simulink model "SSIV_Simulink_Com"  (R2018a)
settings: Solver=FixedStepAuto  StartTime=0.0  StopTime=inf  FixedStep=.015  RelTol=1e-3  EnableMultiTasking=on
libraries: raspberrypilib x24, hdlsllib x21, simulink x11
(part 1 of 2)
settings Model: SimulationMode=external  Creator=domin  LastModifiedBy=domin
settings SolverCC: ConcurrentTasks=on  PositivePriorityOrder=on  AutoInsertRateTranBlk=on
settings DataIOCC: SaveFormat=Array
settings OptimizationCC: EnhancedBackFolding=on  PassReuseOutputArgsThreshold=0  MaxStackSize=64  OptimizeBlockOrder=speed  DifferentSizesBufferReuse=on  OptimizationCustomize=off
settings DebuggingCC: ParameterTunabilityLossMsg=error
settings HardwareCC: ProdBitPerPointer=32  ProdBitPerSizeT=32  ProdBitPerPtrDiffT=32  ProdLargestAtomicInteger=Long  ProdLargestAtomicFloat=Double  ProdWordSize=32  ProdHWDeviceType=ARM Compatible->ARM Cortex  UseEmbeddedCoderFeatures=off  UseSimulinkCoderFeatures=off
settings SFSimCC: MATLABDynamicMemAlloc=off
settings RTWCC: SystemTargetFile=ert.tlc  HardwareBoard=Raspberry Pi  TLCOptions="-aInlineSetEventsForThisBaseRateFcn=TLC_FALSE -aSuppressMultiTaskScheduler=TLC_FALSE  -aRateBasedStepFcn=0"  TemplateMakefile=ert_default_tmf  RTWVerbose=off  Toolchain=GNU GCC Raspberry Pi  BuildConfiguration=Faster Runs
settings CodeAppCC: ForceParamTrailComments=on  OperatorAnnotations=on  MangleLength=10
settings ERTTargetCC: ERTCustomFileBanners=off  SupportContinuousTime=on  SupportNonInlinedSFcns=on  RemoveResetFunc=off  SupportVariableSizeSignals=on  ModelStepFunctionPrototypeControlCompliant=off  ExtMode=on  ExtModeMexArgs='129.65.101.12' 0 17725  ERTSrcFileBannerTemplate=codertarget_code_template.cgt  ERTHdrFileBannerTemplate=codertarget_code_template.cgt  ERTDataSrcFileTemplate=codertarget_code_template.cgt  ERTDataHdrFileTemplate=codertarget_code_template.cgt

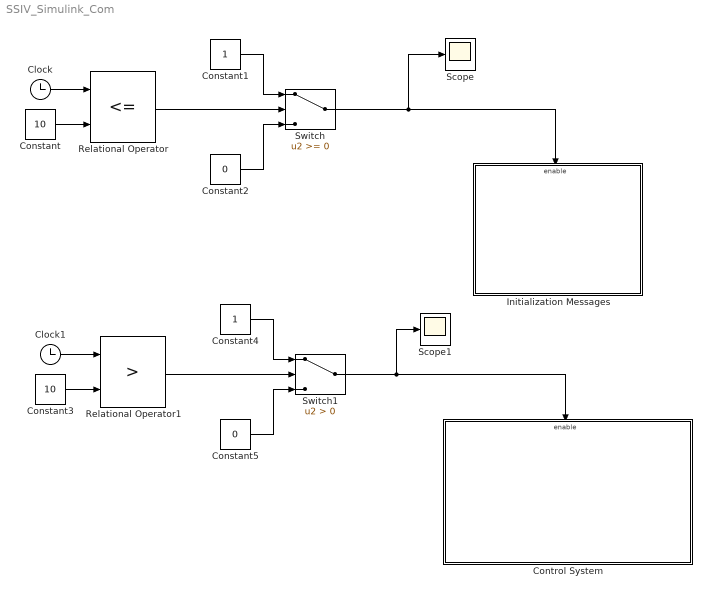
== system SSIV_Simulink_Com ==
  Clock : Clock
  Clock1 : Clock
  Constant : Constant  Value=10
  Constant1 : Constant
  Constant2 : Constant  Value=0
  Constant3 : Constant  Value=10
  Constant4 : Constant
  Constant5 : Constant  Value=0
  Control System : Subsystem
  Initialization Messages : Subsystem
  Relational Operator : RelationalOperator  Operator=<=  OutDataTypeStr=boolean  RndMeth=Simplest
  Relational Operator1 : RelationalOperator  Operator=>  OutDataTypeStr=boolean  RndMeth=Simplest
  Scope : Scope
  Scope1 : Scope
  Switch : Switch
  Switch1 : Switch  Criteria=u2 > Threshold
  wires:
  Clock/1 -> Relational Operator/1
  Constant/1 -> Relational Operator/2
  Relational Operator/1 -> Switch/2
  Constant1/1 -> Switch/1
  Constant2/1 -> Switch/3
  Switch/1 -> Scope/1, Initialization Messages/Enable
  Switch1/1 -> Scope1/1, Control System/Enable
  Constant5/1 -> Switch1/3
  Constant4/1 -> Switch1/1
  Relational Operator1/1 -> Switch1/2
  Constant3/1 -> Relational Operator1/2
  Clock1/1 -> Relational Operator1/1

== system SSIV_Simulink_Com/Control System ==
  Enable : EnablePort
  Const Mot Vel : Constant  Value=50
  SSIV Hardware Communication : Subsystem
  Throttle and Steering Handler : Subsystem
  wires:
  SSIV Hardware Communication/10(radio_throttle) -> Throttle and Steering Handler/1(Inport)
  SSIV Hardware Communication/11(radio_steering) -> Throttle and Steering Handler/3(Inport1)
  Throttle and Steering Handler/1(Throttle RF) -> SSIV Hardware Communication/1(throttle_right_front)
  Throttle and Steering Handler/2(Throttle LF) -> SSIV Hardware Communication/2(throttle_left_front)
  Throttle and Steering Handler/3(Throttle RR) -> SSIV Hardware Communication/3(throttle_right_rear)
  Throttle and Steering Handler/4(Throttle LR) -> SSIV Hardware Communication/4(throttle_left_rear)
  Throttle and Steering Handler/5(Outport) -> SSIV Hardware Communication/5(servo_out)
  Const Mot Vel/1 -> Throttle and Steering Handler/2(Inport2)

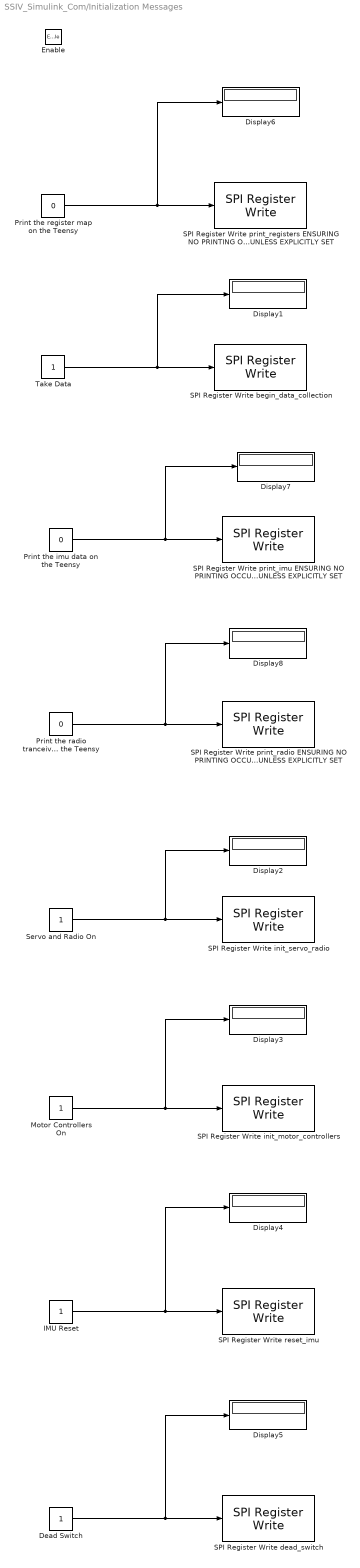
== system SSIV_Simulink_Com/Initialization Messages ==
  Enable : EnablePort
  Dead Switch : Constant  OutDataTypeStr=uint8
  Display{1..8} (8 alike) : Display
      settings: Format=decimal (Stored Integer)
  IMU Reset : Constant  OutDataTypeStr=uint8
  Motor Controllers On : Constant  OutDataTypeStr=uint8
  Print the imu data on the Teensy : Constant  Value=0  OutDataTypeStr=uint8
  Print the radio tranceiver data on the Teensy : Constant  Value=0  OutDataTypeStr=uint8
  Print the register map on the Teensy : Constant  Value=0  OutDataTypeStr=uint8
  SPI Register Write begin_data_collection : raspberrypilib/SPI Register Write  BoardProperty=Pi 3 Model B  SPIModule=uint32(0)  Mode=Master  BusSpeed=1000000  Pin=SPI0_CE1  FirstBitToTransfer=Most significant bit (MSB)  ClockMode=0  BlockFunction=Write  RegisterAddress=1  OutputDataType=int8  OutputDataLength=1
      settings: SourceProductName=Simulink Support Package for Raspberry Pi Hardware  SourceProductBaseCode=RASPPI
  SPI Register Write dead_switch : raspberrypilib/SPI Register Write  BoardProperty=Pi 3 Model B  SPIModule=uint32(0)  Mode=Master  BusSpeed=1000000  Pin=SPI0_CE1  FirstBitToTransfer=Most significant bit (MSB)  ClockMode=0  BlockFunction=Write  RegisterAddress=7  OutputDataType=int8  OutputDataLength=1
      settings: SourceProductName=Simulink Support Package for Raspberry Pi Hardware  SourceProductBaseCode=RASPPI
  SPI Register Write init_motor_controllers : raspberrypilib/SPI Register Write  BoardProperty=Pi 3 Model B  SPIModule=uint32(0)  Mode=Master  BusSpeed=1000000  Pin=SPI0_CE1  FirstBitToTransfer=Most significant bit (MSB)  ClockMode=0  BlockFunction=Write  RegisterAddress=5  OutputDataType=int8  OutputDataLength=1
      settings: SourceProductName=Simulink Support Package for Raspberry Pi Hardware  SourceProductBaseCode=RASPPI
  SPI Register Write init_servo_radio : raspberrypilib/SPI Register Write  BoardProperty=Pi 3 Model B  SPIModule=uint32(0)  Mode=Master  BusSpeed=1000000  Pin=SPI0_CE1  FirstBitToTransfer=Most significant bit (MSB)  ClockMode=0  BlockFunction=Write  RegisterAddress=4  OutputDataType=int8  OutputDataLength=1
      settings: SourceProductName=Simulink Support Package for Raspberry Pi Hardware  SourceProductBaseCode=RASPPI
  SPI Register Write print_imu ENSURING NO PRINTING OCCURS DURING DYNAMIC OP UNLESS EXPLICITLY SET : raspberrypilib/SPI Register Write  BoardProperty=Pi 3 Model B  SPIModule=uint32(0)  Mode=Master  BusSpeed=1000000  Pin=SPI0_CE1  FirstBitToTransfer=Most significant bit (MSB)  ClockMode=0  BlockFunction=Write  RegisterAddress=2  OutputDataType=int8  OutputDataLength=1
      settings: SourceProductName=Simulink Support Package for Raspberry Pi Hardware  SourceProductBaseCode=RASPPI
  SPI Register Write print_radio ENSURING NO PRINTING OCCURS DURING DYNAMIC OP UNLESS EXPLICITLY SET : raspberrypilib/SPI Register Write  BoardProperty=Pi 3 Model B  SPIModule=uint32(0)  Mode=Master  BusSpeed=1000000  Pin=SPI0_CE1  FirstBitToTransfer=Most significant bit (MSB)  ClockMode=0  BlockFunction=Write  RegisterAddress=3  OutputDataType=int8  OutputDataLength=1
      settings: SourceProductName=Simulink Support Package for Raspberry Pi Hardware  SourceProductBaseCode=RASPPI
  SPI Register Write print_registers ENSURING NO PRINTING OCCURS DURING DYNAMIC OP UNLESS EXPLICITLY SET : raspberrypilib/SPI Register Write  BoardProperty=Pi 3 Model B  SPIModule=uint32(0)  Mode=Master  BusSpeed=1000000  Pin=SPI0_CE1  FirstBitToTransfer=Most significant bit (MSB)  ClockMode=0  BlockFunction=Write  RegisterAddress=0  OutputDataType=int8  OutputDataLength=1
      settings: SourceProductName=Simulink Support Package for Raspberry Pi Hardware  SourceProductBaseCode=RASPPI
  SPI Register Write reset_imu : raspberrypilib/SPI Register Write  BoardProperty=Pi 3 Model B  SPIModule=uint32(0)  Mode=Master  BusSpeed=1000000  Pin=SPI0_CE1  FirstBitToTransfer=Most significant bit (MSB)  ClockMode=0  BlockFunction=Write  RegisterAddress=6  OutputDataType=int8  OutputDataLength=1
      settings: SourceProductName=Simulink Support Package for Raspberry Pi Hardware  SourceProductBaseCode=RASPPI
  Servo and Radio On : Constant  OutDataTypeStr=uint8
  Take Data : Constant  OutDataTypeStr=uint8
  wires:
  Take Data/1 -> Display1/1, SPI Register Write begin_data_collection/1
  Servo and Radio On/1 -> SPI Register Write init_servo_radio/1, Display2/1
  Motor Controllers On/1 -> Display3/1, SPI Register Write init_motor_controllers/1
  IMU Reset/1 -> SPI Register Write reset_imu/1, Display4/1
  Dead Switch/1 -> Display5/1, SPI Register Write dead_switch/1
  Print the register map on the Teensy/1 -> SPI Register Write print_registers ENSURING NO PRINTING OCCURS DURING DYNAMIC OP UNLESS EXPLICITLY SET/1, Display6/1
  Print the imu data on the Teensy/1 -> SPI Register Write print_imu ENSURING NO PRINTING OCCURS DURING DYNAMIC OP UNLESS EXPLICITLY SET/1, Display7/1
  Print the radio tranceiver data on the Teensy/1 -> Display8/1, SPI Register Write print_radio ENSURING NO PRINTING OCCURS DURING DYNAMIC OP UNLESS EXPLICITLY SET/1

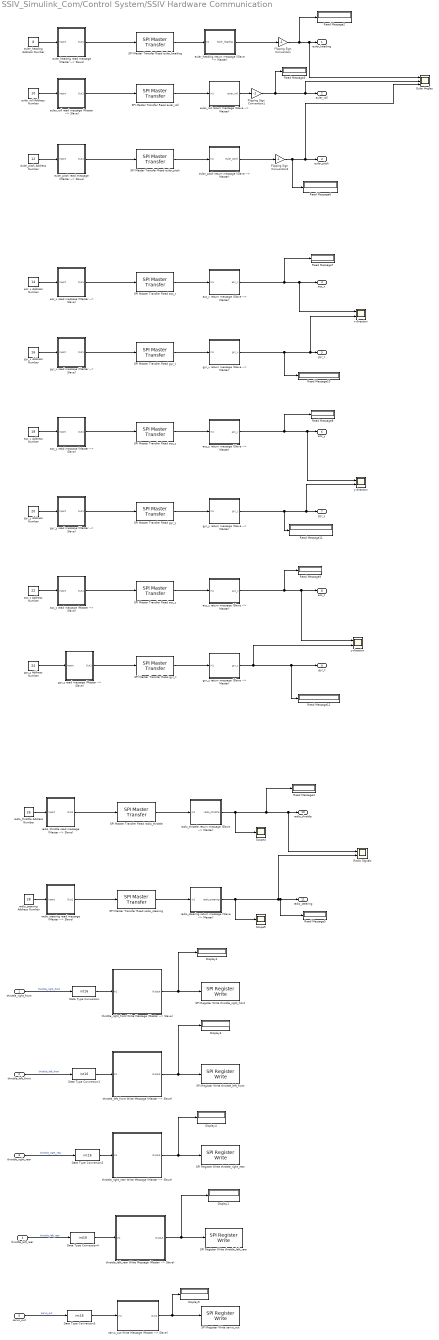
== system SSIV_Simulink_Com/Control System/SSIV Hardware Communication ==
  throttle_right_front : Inport
  throttle_left_front : Inport  Port=2
  throttle_right_rear : Inport  Port=3
  throttle_left_rear : Inport  Port=4
  servo_out : Inport  Port=5
  Data Type Conversion{,1..4} (5 alike) : DataTypeConversion  OutDataTypeStr=int16  RndMeth=Nearest
  Display{1..5} (5 alike) : Display
      settings: Format=decimal (Stored Integer)
  Euler Angles : Scope  NumInputPorts=3
  Flipping Sign Convention : Gain  Gain=-1
  Flipping Sign Convention1 : Gain  Gain=-1
  Flipping Sign Convention2 : Gain  Gain=-1
  Radio SIgnals : Scope  NumInputPorts=2
  Read Message{2..12} (11 alike) : Display
      settings: Format=decimal (Stored Integer)
  SPI Master Transfer Read acc_x : raspberrypilib/SPI Master Transfer  BoardProperty=Pi 3 Model B  SPIModule=uint32(0)  Mode=Master  BusSpeed=1000000  Pin=SPI0_CE1  FirstBitToTransfer=Most significant bit (MSB)  ClockMode=0  BlockFunction=Transfer  RegisterAddress=0  OutputDataType=int8  OutputDataLength=1
      settings: SourceProductName=Simulink Support Package for Raspberry Pi Hardware  SourceProductBaseCode=RASPPI
  SPI Master Transfer Read acc_y : raspberrypilib/SPI Master Transfer  BoardProperty=Pi 3 Model B  SPIModule=uint32(0)  Mode=Master  BusSpeed=1000000  Pin=SPI0_CE1  FirstBitToTransfer=Most significant bit (MSB)  ClockMode=0  BlockFunction=Transfer  RegisterAddress=0  OutputDataType=int8  OutputDataLength=1
      settings: SourceProductName=Simulink Support Package for Raspberry Pi Hardware  SourceProductBaseCode=RASPPI
  SPI Master Transfer Read acc_z : raspberrypilib/SPI Master Transfer  BoardProperty=Pi 3 Model B  SPIModule=uint32(0)  Mode=Master  BusSpeed=1000000  Pin=SPI0_CE1  FirstBitToTransfer=Most significant bit (MSB)  ClockMode=0  BlockFunction=Transfer  RegisterAddress=0  OutputDataType=int8  OutputDataLength=1
      settings: SourceProductName=Simulink Support Package for Raspberry Pi Hardware  SourceProductBaseCode=RASPPI
  SPI Master Transfer Read euler_heading : raspberrypilib/SPI Master Transfer  BoardProperty=Pi 3 Model B  SPIModule=uint32(0)  Mode=Master  BusSpeed=1000000  Pin=SPI0_CE1  FirstBitToTransfer=Most significant bit (MSB)  ClockMode=0  BlockFunction=Transfer  RegisterAddress=0  OutputDataType=int8  OutputDataLength=1
      settings: SourceProductName=Simulink Support Package for Raspberry Pi Hardware  SourceProductBaseCode=RASPPI
  SPI Master Transfer Read euler_pitch : raspberrypilib/SPI Master Transfer  BoardProperty=Pi 3 Model B  SPIModule=uint32(0)  Mode=Master  BusSpeed=1000000  Pin=SPI0_CE1  FirstBitToTransfer=Most significant bit (MSB)  ClockMode=0  BlockFunction=Transfer  RegisterAddress=0  OutputDataType=int8  OutputDataLength=1
      settings: SourceProductName=Simulink Support Package for Raspberry Pi Hardware  SourceProductBaseCode=RASPPI
  SPI Master Transfer Read euler_roll : raspberrypilib/SPI Master Transfer  BoardProperty=Pi 3 Model B  SPIModule=uint32(0)  Mode=Master  BusSpeed=1000000  Pin=SPI0_CE1  FirstBitToTransfer=Most significant bit (MSB)  ClockMode=0  BlockFunction=Transfer  RegisterAddress=0  OutputDataType=int8  OutputDataLength=1
      settings: SourceProductName=Simulink Support Package for Raspberry Pi Hardware  SourceProductBaseCode=RASPPI
  SPI Master Transfer Read gyr_x : raspberrypilib/SPI Master Transfer  BoardProperty=Pi 3 Model B  SPIModule=uint32(0)  Mode=Master  BusSpeed=1000000  Pin=SPI0_CE1  FirstBitToTransfer=Most significant bit (MSB)  ClockMode=0  BlockFunction=Transfer  RegisterAddress=0  OutputDataType=int8  OutputDataLength=1
      settings: SourceProductName=Simulink Support Package for Raspberry Pi Hardware  SourceProductBaseCode=RASPPI
  SPI Master Transfer Read gyr_y : raspberrypilib/SPI Master Transfer  BoardProperty=Pi 3 Model B  SPIModule=uint32(0)  Mode=Master  BusSpeed=1000000  Pin=SPI0_CE1  FirstBitToTransfer=Most significant bit (MSB)  ClockMode=0  BlockFunction=Transfer  RegisterAddress=0  OutputDataType=int8  OutputDataLength=1
      settings: SourceProductName=Simulink Support Package for Raspberry Pi Hardware  SourceProductBaseCode=RASPPI
  SPI Master Transfer Read gyr_z : raspberrypilib/SPI Master Transfer  BoardProperty=Pi 3 Model B  SPIModule=uint32(0)  Mode=Master  BusSpeed=1000000  Pin=SPI0_CE1  FirstBitToTransfer=Most significant bit (MSB)  ClockMode=0  BlockFunction=Transfer  RegisterAddress=0  OutputDataType=int8  OutputDataLength=1
      settings: SourceProductName=Simulink Support Package for Raspberry Pi Hardware  SourceProductBaseCode=RASPPI
  SPI Master Transfer Read radio_steering : raspberrypilib/SPI Master Transfer  BoardProperty=Pi 3 Model B  SPIModule=uint32(0)  Mode=Master  BusSpeed=1000000  Pin=SPI0_CE1  FirstBitToTransfer=Most significant bit (MSB)  ClockMode=0  BlockFunction=Transfer  RegisterAddress=0  OutputDataType=int8  OutputDataLength=1
      settings: SourceProductName=Simulink Support Package for Raspberry Pi Hardware  SourceProductBaseCode=RASPPI
  SPI Master Transfer Read radio_throttle : raspberrypilib/SPI Master Transfer  BoardProperty=Pi 3 Model B  SPIModule=uint32(0)  Mode=Master  BusSpeed=1000000  Pin=SPI0_CE1  FirstBitToTransfer=Most significant bit (MSB)  ClockMode=0  BlockFunction=Transfer  RegisterAddress=0  OutputDataType=int8  OutputDataLength=1
      settings: SourceProductName=Simulink Support Package for Raspberry Pi Hardware  SourceProductBaseCode=RASPPI
  "SPI Register Write servo_out " : raspberrypilib/SPI Register Write  BoardProperty=Pi 3 Model B  SPIModule=uint32(0)  Mode=Master  BusSpeed=1000000  Pin=SPI0_CE1  FirstBitToTransfer=Most significant bit (MSB)  ClockMode=0  BlockFunction=Write  RegisterAddress=38  OutputDataType=int8  OutputDataLength=1
      settings: SourceProductName=Simulink Support Package for Raspberry Pi Hardware  SourceProductBaseCode=RASPPI
  SPI Register Write throttle_left_front : raspberrypilib/SPI Register Write  BoardProperty=Pi 3 Model B  SPIModule=uint32(0)  Mode=Master  BusSpeed=1000000  Pin=SPI0_CE1  FirstBitToTransfer=Most significant bit (MSB)  ClockMode=0  BlockFunction=Write  RegisterAddress=32  OutputDataType=int8  OutputDataLength=1
      settings: SourceProductName=Simulink Support Package for Raspberry Pi Hardware  SourceProductBaseCode=RASPPI
  SPI Register Write throttle_left_rear : raspberrypilib/SPI Register Write  BoardProperty=Pi 3 Model B  SPIModule=uint32(0)  Mode=Master  BusSpeed=1000000  Pin=SPI0_CE1  FirstBitToTransfer=Most significant bit (MSB)  ClockMode=0  BlockFunction=Write  RegisterAddress=36  OutputDataType=int8  OutputDataLength=1
      settings: SourceProductName=Simulink Support Package for Raspberry Pi Hardware  SourceProductBaseCode=RASPPI
  SPI Register Write throttle_right_front : raspberrypilib/SPI Register Write  BoardProperty=Pi 3 Model B  SPIModule=uint32(0)  Mode=Master  BusSpeed=1000000  Pin=SPI0_CE1  FirstBitToTransfer=Most significant bit (MSB)  ClockMode=0  BlockFunction=Write  RegisterAddress=30  OutputDataType=int8  OutputDataLength=1
      settings: SourceProductName=Simulink Support Package for Raspberry Pi Hardware  SourceProductBaseCode=RASPPI
  SPI Register Write throttle_right_rear : raspberrypilib/SPI Register Write  BoardProperty=Pi 3 Model B  SPIModule=uint32(0)  Mode=Master  BusSpeed=1000000  Pin=SPI0_CE1  FirstBitToTransfer=Most significant bit (MSB)  ClockMode=0  BlockFunction=Write  RegisterAddress=34  OutputDataType=int8  OutputDataLength=1
      settings: SourceProductName=Simulink Support Package for Raspberry Pi Hardware  SourceProductBaseCode=RASPPI
  Scope4 : Scope
  Scope5 : Scope
  acc_x Address Number : Constant  Value=14  OutDataTypeStr=uint8
  acc_x read message (Master --> Slave) : Subsystem
  acc_x return message (Slave --> Master) : Subsystem
  acc_y Address Number : Constant  Value=18  OutDataTypeStr=uint8
  acc_y read message (Master --> Slave) : Subsystem
  acc_y return message (Slave --> Master) : Subsystem
  acc_z Address Number : Constant  Value=22  OutDataTypeStr=uint8
  acc_z read message (Master --> Slave) : Subsystem
  acc_z return message (Slave --> Master) : Subsystem
  euler_heading Address Number : Constant  Value=8  OutDataTypeStr=uint8
  euler_heading read message (Master --> Slave) : Subsystem
  euler_heading return message (Slave --> Master) : Subsystem
  euler_pitch Address Number : Constant  Value=12  OutDataTypeStr=uint8
  euler_pitch read message (Master --> Slave) : Subsystem
  euler_pitch return message (Slave --> Master) : Subsystem
  euler_roll Address Number : Constant  Value=10  OutDataTypeStr=uint8
  euler_roll read message (Master --> Slave) : Subsystem
  euler_roll return message (Slave --> Master) : Subsystem
  gyr_x Address Number : Constant  Value=16  OutDataTypeStr=uint8
  gyr_x read message (Master --> Slave) : Subsystem
  gyr_x return message (Slave --> Master) : Subsystem
  "gyr_y Address Number " : Constant  Value=20  OutDataTypeStr=uint8
  gyr_y read message (Master --> Slave) : Subsystem
  gyr_y return message (Slave --> Master) : Subsystem
  gyr_z Address Number : Constant  Value=24  OutDataTypeStr=uint8
  gyr_z read message (Master --> Slave) : Subsystem
  gyr_z return message (Slave --> Master) : Subsystem
  radio_steering Address Number : Constant  Value=28  OutDataTypeStr=uint8
  radio_steering read message (Master --> Slave) : Subsystem
  radio_steering return message (Slave --> Master) : Subsystem
  "radio_throttle Address Number " : Constant  Value=26  OutDataTypeStr=uint8
  radio_throttle read message (Master --> Slave) : Subsystem
  radio_throttle return message (Slave --> Master) : Subsystem
  servo_out Write Message (Master --> Slave) : Subsystem
  throttle_left_front Write Message (Master --> Slave) : Subsystem
  throttle_left_rear Write Message (Master --> Slave) : Subsystem
  throttle_right_front Write Message (Master --> Slave) : Subsystem
  throttle_right_rear Write Message (Master --> Slave) : Subsystem
  x-direction : Scope  NumInputPorts=2
  y-direction : Scope  NumInputPorts=2
  z-direction : Scope  NumInputPorts=2
  euler_heading : Outport
  euler_roll : Outport  Port=2
  euler_pitch : Outport  Port=3
  acc_x : Outport  Port=4
  gyr_x : Outport  Port=5
  acc_y : Outport  Port=6
  gyr_y : Outport  Port=7
  acc_z : Outport  Port=8
  gyr_z : Outport  Port=9
  radio_throttle : Outport  Port=10
  radio_steering : Outport  Port=11
  wires:
  euler_heading read message (Master --> Slave)/1(Out1) -> SPI Master Transfer Read euler_heading/1
  euler_heading return message (Slave --> Master)/1(euler_heading) -> Flipping Sign Convention/1
  SPI Master Transfer Read euler_heading/1 -> euler_heading return message (Slave --> Master)/1(In1)
  throttle_left_rear Write Message (Master --> Slave)/1(Output) -> Display1/1, SPI Register Write throttle_left_rear/1
  throttle_left_rear/1 -> Data Type Conversion4/1  "throttle_left_rear"
  SPI Master Transfer Read radio_throttle/1 -> radio_throttle return message (Slave --> Master)/1(In1)
  radio_throttle read message (Master --> Slave)/1(Out1) -> SPI Master Transfer Read radio_throttle/1
  radio_throttle return message (Slave --> Master)/1(radio_throttle) -> Read Message4/1, Radio SIgnals/1, radio_throttle/1, Scope4/1
  radio_steering return message (Slave --> Master)/1(radio_steering) -> Read Message5/1, radio_steering/1, Radio SIgnals/2, Scope5/1
  radio_steering read message (Master --> Slave)/1(Out1) -> SPI Master Transfer Read radio_steering/1
  SPI Master Transfer Read radio_steering/1 -> radio_steering return message (Slave --> Master)/1(In1)
  servo_out/1 -> Data Type Conversion3/1  "servo_out"
  servo_out Write Message (Master --> Slave)/1(Out1) -> Display5/1, "SPI Register Write servo_out "/1
  acc_x return message (Slave --> Master)/1(acc_x) -> Read Message7/1, x-direction/1, acc_x/1
  SPI Master Transfer Read acc_x/1 -> acc_x return message (Slave --> Master)/1(In1)
  acc_x read message (Master --> Slave)/1(Out1) -> SPI Master Transfer Read acc_x/1
  acc_y read message (Master --> Slave)/1(Out1) -> SPI Master Transfer Read acc_y/1
  SPI Master Transfer Read acc_y/1 -> acc_y return message (Slave --> Master)/1(In1)
  acc_y return message (Slave --> Master)/1(acc_y) -> y-direction/1, acc_y/1, Read Message8/1
  acc_z return message (Slave --> Master)/1(acc_z) -> z-direction/1, acc_z/1, Read Message9/1
  SPI Master Transfer Read acc_z/1 -> acc_z return message (Slave --> Master)/1(In1)
  acc_z read message (Master --> Slave)/1(Out1) -> SPI Master Transfer Read acc_z/1
  gyr_z read message (Master --> Slave)/1(Out1) -> SPI Master Transfer Read gyr_z/1
  SPI Master Transfer Read gyr_z/1 -> gyr_z return message (Slave --> Master)/1(In1)
  gyr_z return message (Slave --> Master)/1(gyr_z) -> z-direction/2, gyr_z/1, Read Message12/1
  gyr_y return message (Slave --> Master)/1(gyr_y) -> Read Message11/1, y-direction/2, gyr_y/1
  SPI Master Transfer Read gyr_y/1 -> gyr_y return message (Slave --> Master)/1(In1)
  gyr_y read message (Master --> Slave)/1(Out1) -> SPI Master Transfer Read gyr_y/1
  gyr_x read message (Master --> Slave)/1(Out1) -> SPI Master Transfer Read gyr_x/1
  SPI Master Transfer Read gyr_x/1 -> gyr_x return message (Slave --> Master)/1(In1)
  gyr_x return message (Slave --> Master)/1(gyr_x) -> x-direction/2, gyr_x/1, Read Message10/1
  throttle_right_front/1 -> Data Type Conversion/1  "throttle_right_front"
  throttle_right_front Write Message (Master --> Slave)/1(Output) -> SPI Register Write throttle_right_front/1, Display2/1
  throttle_right_rear Write Message (Master --> Slave)/1(Output) -> Display4/1, SPI Register Write throttle_right_rear/1
  throttle_right_rear/1 -> Data Type Conversion2/1  "throttle_right_rear"
  throttle_left_front/1 -> Data Type Conversion1/1  "throttle_left_front"
  throttle_left_front Write Message (Master --> Slave)/1(Output) -> SPI Register Write throttle_left_front/1, Display3/1
  Data Type Conversion/1 -> throttle_right_front Write Message (Master --> Slave)/1(In1)
  Data Type Conversion1/1 -> throttle_left_front Write Message (Master --> Slave)/1(In1)
  Data Type Conversion2/1 -> throttle_right_rear Write Message (Master --> Slave)/1(In1)
  Data Type Conversion3/1 -> servo_out Write Message (Master --> Slave)/1(In1)
  Data Type Conversion4/1 -> throttle_left_rear Write Message (Master --> Slave)/1(In1)
  "radio_throttle Address Number "/1 -> radio_throttle read message (Master --> Slave)/1(Inport)
  gyr_z Address Number/1 -> gyr_z read message (Master --> Slave)/1(Inport)
  "gyr_y Address Number "/1 -> gyr_y read message (Master --> Slave)/1(Inport)
  gyr_x Address Number/1 -> gyr_x read message (Master --> Slave)/1(Inport)
  acc_z Address Number/1 -> acc_z read message (Master --> Slave)/1(Inport)
  acc_y Address Number/1 -> acc_y read message (Master --> Slave)/1(Inport)
  acc_x Address Number/1 -> acc_x read message (Master --> Slave)/1(Inport)
  euler_heading Address Number/1 -> euler_heading read message (Master --> Slave)/1(Inport)
  radio_steering Address Number/1 -> radio_steering read message (Master --> Slave)/1(Inport)
  SPI Master Transfer Read euler_roll/1 -> euler_roll return message (Slave --> Master)/1(In1)
  euler_roll Address Number/1 -> euler_roll read message (Master --> Slave)/1(Inport)
  euler_roll read message (Master --> Slave)/1(Out1) -> SPI Master Transfer Read euler_roll/1
  euler_roll return message (Slave --> Master)/1(euler_roll) -> Flipping Sign Convention1/1
  euler_pitch return message (Slave --> Master)/1(euler_pitch) -> Flipping Sign Convention2/1
  euler_pitch Address Number/1 -> euler_pitch read message (Master --> Slave)/1(Inport)
  SPI Master Transfer Read euler_pitch/1 -> euler_pitch return message (Slave --> Master)/1(In1)
  euler_pitch read message (Master --> Slave)/1(Out1) -> SPI Master Transfer Read euler_pitch/1
  Flipping Sign Convention/1 -> Read Message2/1, Euler Angles/1, euler_heading/1
  Flipping Sign Convention1/1 -> Read Message3/1, Euler Angles/2, euler_roll/1
  Flipping Sign Convention2/1 -> Read Message6/1, Euler Angles/3, euler_pitch/1

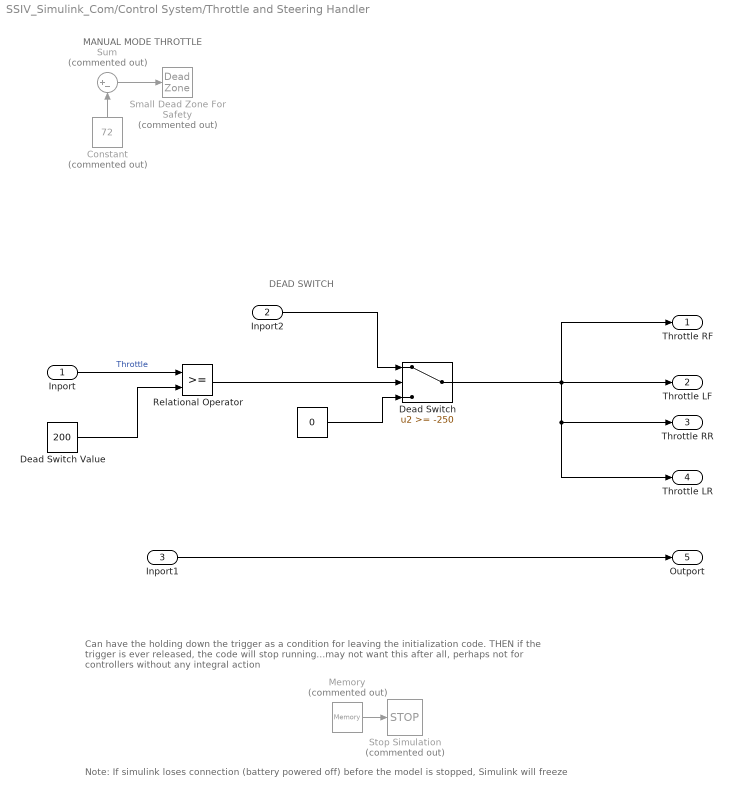
== system SSIV_Simulink_Com/Control System/Throttle and Steering Handler ==
  note: MANUAL MODE THROTTLE
  note: DEAD SWITCH
  note: Note: If simulink loses connection (battery powered off) before the model is stopped, Simulink will freeze
  note: Can have the holding down the trigger as a condition for leaving the initialization code. THEN if the trigger is ever released, the code will stop running...may not want this after all, perhaps not for controllers without any integral action
  Inport : Inport
  Inport2 : Inport  Port=2
  Inport1 : Inport  Port=3
  " " : Constant  Value=0
  Constant : Constant  Commented=on  Value=72
  Dead Switch : Switch  Threshold=-250
  Dead Switch Value : Constant  Value=200
  Memory : Memory  Commented=on
  Relational Operator : RelationalOperator  RndMeth=Simplest
  Small Dead Zone For Safety : DeadZone  Commented=on  LowerValue=-10  UpperValue=10
  Stop Simulation : Stop  Commented=on
  Sum : Sum  Commented=on  Inputs=|+-
  Throttle RF : Outport
  Throttle LF : Outport  Port=2
  Throttle RR : Outport  Port=3
  Throttle LR : Outport  Port=4
  Outport : Outport  Port=5
  wires:
  Inport1/1 -> Outport/1
  " "/1 -> Dead Switch/3
  Inport2/1 -> Dead Switch/1
  Relational Operator/1 -> Dead Switch/2
  Dead Switch/1 -> Throttle LF/1, Throttle LR/1, Throttle RR/1, Throttle RF/1
  Inport/1 -> Relational Operator/1  "Throttle"
  Memory/1 -> Stop Simulation/1
  Dead Switch Value/1 -> Relational Operator/2
  Constant/1 -> Sum/2
  Sum/1 -> Small Dead Zone For Safety/1

== system SSIV_Simulink_Com/Control System/SSIV Hardware Communication/acc_x read message (Master --> Slave) ==
  Inport : Inport
  Mux : Mux
      settings: DisplayOption=signals
  Read Bit Set : simulink/Logic and Bit Operations/Bit Set  iBit=7
      settings: SourceProductName=Simulink  SourceProductBaseCode=SL
  uint8_t 1 : Constant  OutDataTypeStr=uint8
  uint8_t 2 : Constant  OutDataTypeStr=uint8
  uint8_t 3 : Constant  OutDataTypeStr=uint8
  Out1 : Outport
  wires:
  Read Bit Set/1 -> Mux/1  "Addres/RW Byte acc_x Teensy Status will be returned here"
  uint8_t 1/1 -> Mux/2  "Junk will be returned here"
  Inport/1 -> Read Bit Set/1
  uint8_t 3/1 -> Mux/4  "Byte 1 will be returned here"
  Mux/1 -> Out1/1
  uint8_t 2/1 -> Mux/3  "Byte 0 will be returned here"

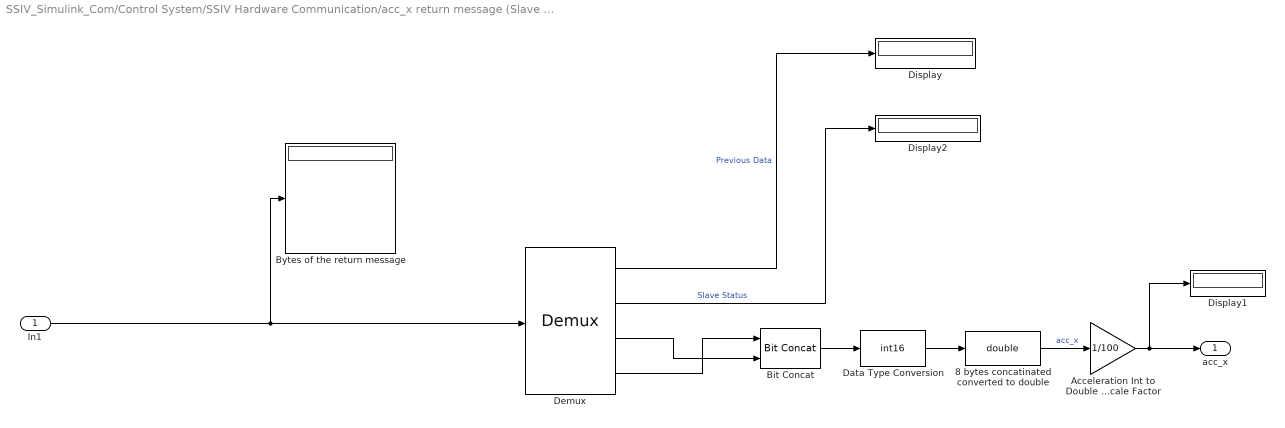
== system SSIV_Simulink_Com/Control System/SSIV Hardware Communication/acc_x return message (Slave --> Master) ==
  In1 : Inport
  8 bytes concatinated converted to double : DataTypeConversion  OutDataTypeStr=double  RndMeth=Nearest
  Acceleration Int to Double Scale Factor : Gain  Gain=1/100
  Bit Concat : hdlsllib/Logic and Bit Operations/Bit Concat  numInputs=2
      settings: SourceProductName=HDL Coder  SourceProductBaseCode=HD
  Bytes of the return message : Display
      settings: Format=decimal (Stored Integer)
  Data Type Conversion : DataTypeConversion  OutDataTypeStr=int16  RndMeth=Nearest
  Demux : Demux
  Display : Display
      settings: Format=binary (Stored Integer)
  Display1 : Display
      settings: Format=decimal (Stored Integer)
  Display2 : Display
      settings: Format=binary (Stored Integer)
  acc_x : Outport
  wires:
  8 bytes concatinated converted to double/1 -> Acceleration Int to Double Scale Factor/1  "acc_x"
  Demux/2 -> Display2/1  "Slave Status"
  Demux/1 -> Display/1  "Previous Data"
  In1/1 -> Bytes of the return message/1, Demux/1
  Bit Concat/1 -> Data Type Conversion/1
  Demux/4 -> Bit Concat/1
  Demux/3 -> Bit Concat/2
  Acceleration Int to Double Scale Factor/1 -> Display1/1, acc_x/1
  Data Type Conversion/1 -> 8 bytes concatinated converted to double/1

== system SSIV_Simulink_Com/Control System/SSIV Hardware Communication/acc_y read message (Master --> Slave) ==
  Inport : Inport
  Mux : Mux
      settings: DisplayOption=signals
  Read Bit Set : simulink/Logic and Bit Operations/Bit Set  iBit=7
      settings: SourceProductName=Simulink  SourceProductBaseCode=SL
  uint8_t 1 : Constant  OutDataTypeStr=uint8
  uint8_t 2 : Constant  OutDataTypeStr=uint8
  uint8_t 3 : Constant  OutDataTypeStr=uint8
  Out1 : Outport
  wires:
  uint8_t 2/1 -> Mux/3  "Byte 0 will be returned here"
  Mux/1 -> Out1/1
  uint8_t 3/1 -> Mux/4  "Byte 1 will be returned here"
  Inport/1 -> Read Bit Set/1
  uint8_t 1/1 -> Mux/2  "Junk will be returned here"
  Read Bit Set/1 -> Mux/1  "Addres/RW Byte acc_y Teensy Status will be returned here"

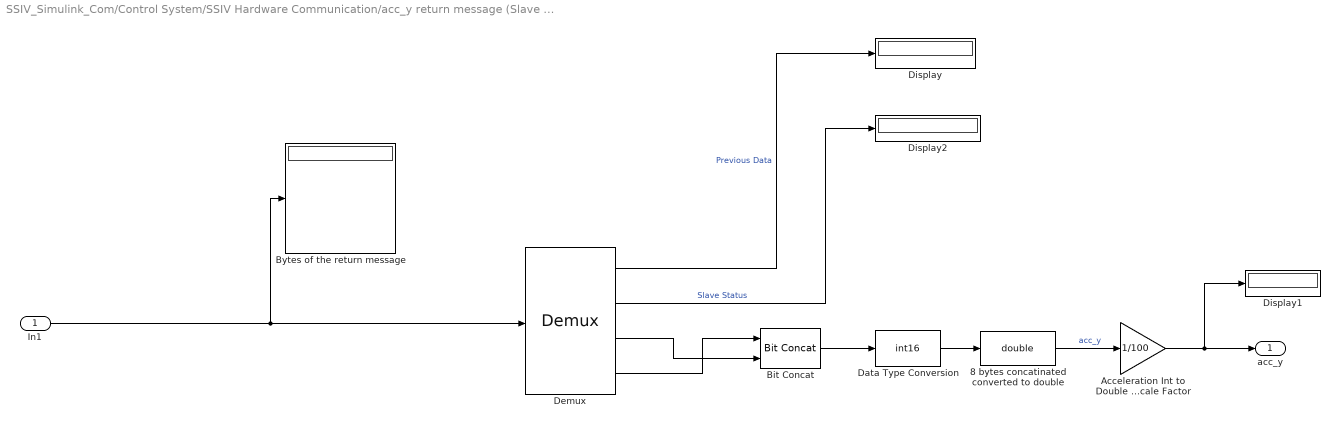
== system SSIV_Simulink_Com/Control System/SSIV Hardware Communication/acc_y return message (Slave --> Master) ==
  In1 : Inport
  8 bytes concatinated converted to double : DataTypeConversion  OutDataTypeStr=double  RndMeth=Nearest
  Acceleration Int to Double Scale Factor : Gain  Gain=1/100
  Bit Concat : hdlsllib/Logic and Bit Operations/Bit Concat  numInputs=2
      settings: SourceProductName=HDL Coder  SourceProductBaseCode=HD
  Bytes of the return message : Display
      settings: Format=decimal (Stored Integer)
  Data Type Conversion : DataTypeConversion  OutDataTypeStr=int16  RndMeth=Nearest
  Demux : Demux
  Display : Display
      settings: Format=binary (Stored Integer)
  Display1 : Display
      settings: Format=decimal (Stored Integer)
  Display2 : Display
      settings: Format=binary (Stored Integer)
  acc_y : Outport
  wires:
  Acceleration Int to Double Scale Factor/1 -> acc_y/1, Display1/1
  Demux/3 -> Bit Concat/2
  Demux/4 -> Bit Concat/1
  Bit Concat/1 -> Data Type Conversion/1
  In1/1 -> Demux/1, Bytes of the return message/1
  Demux/1 -> Display/1  "Previous Data"
  Demux/2 -> Display2/1  "Slave Status"
  8 bytes concatinated converted to double/1 -> Acceleration Int to Double Scale Factor/1  "acc_y"
  Data Type Conversion/1 -> 8 bytes concatinated converted to double/1

== system SSIV_Simulink_Com/Control System/SSIV Hardware Communication/acc_z read message (Master --> Slave) ==
  Inport : Inport
  Mux : Mux
      settings: DisplayOption=signals
  Read Bit Set : simulink/Logic and Bit Operations/Bit Set  iBit=7
      settings: SourceProductName=Simulink  SourceProductBaseCode=SL
  uint8_t 1 : Constant  OutDataTypeStr=uint8
  uint8_t 2 : Constant  OutDataTypeStr=uint8
  uint8_t 3 : Constant  OutDataTypeStr=uint8
  Out1 : Outport
  wires:
  Read Bit Set/1 -> Mux/1  "Addres/RW Byte acc_y Teensy Status will be returned here"
  uint8_t 1/1 -> Mux/2  "Junk will be returned here"
  Inport/1 -> Read Bit Set/1
  uint8_t 3/1 -> Mux/4  "Byte 1 will be returned here"
  Mux/1 -> Out1/1
  uint8_t 2/1 -> Mux/3  "Byte 0 will be returned here"

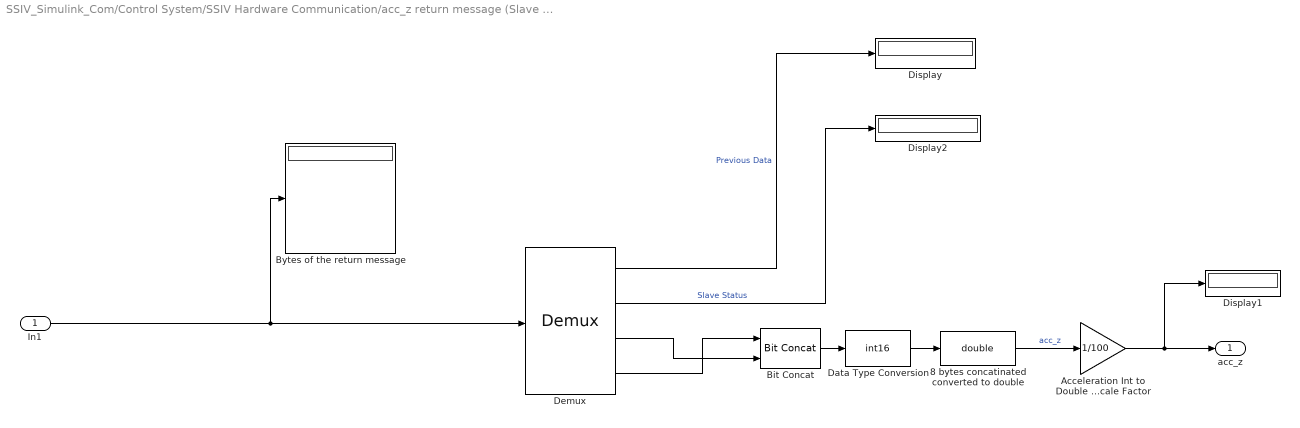
== system SSIV_Simulink_Com/Control System/SSIV Hardware Communication/acc_z return message (Slave --> Master) ==
  In1 : Inport
  8 bytes concatinated converted to double : DataTypeConversion  OutDataTypeStr=double  RndMeth=Nearest
  Acceleration Int to Double Scale Factor : Gain  Gain=1/100
  Bit Concat : hdlsllib/Logic and Bit Operations/Bit Concat  numInputs=2
      settings: SourceProductName=HDL Coder  SourceProductBaseCode=HD
  Bytes of the return message : Display
      settings: Format=decimal (Stored Integer)
  Data Type Conversion : DataTypeConversion  OutDataTypeStr=int16  RndMeth=Nearest
  Demux : Demux
  Display : Display
      settings: Format=binary (Stored Integer)
  Display1 : Display
      settings: Format=decimal (Stored Integer)
  Display2 : Display
      settings: Format=binary (Stored Integer)
  acc_z : Outport
  wires:
  8 bytes concatinated converted to double/1 -> Acceleration Int to Double Scale Factor/1  "acc_z"
  Demux/2 -> Display2/1  "Slave Status"
  Demux/1 -> Display/1  "Previous Data"
  In1/1 -> Bytes of the return message/1, Demux/1
  Bit Concat/1 -> Data Type Conversion/1
  Demux/4 -> Bit Concat/1
  Demux/3 -> Bit Concat/2
  Acceleration Int to Double Scale Factor/1 -> Display1/1, acc_z/1
  Data Type Conversion/1 -> 8 bytes concatinated converted to double/1

== system SSIV_Simulink_Com/Control System/SSIV Hardware Communication/euler_heading read message (Master --> Slave) ==
  Inport : Inport
  Mux : Mux
      settings: DisplayOption=signals
  Read Bit Set : simulink/Logic and Bit Operations/Bit Set  iBit=7
      settings: SourceProductName=Simulink  SourceProductBaseCode=SL
  uint8_t  1 : Constant  OutDataTypeStr=uint8
  uint8_t  2 : Constant  OutDataTypeStr=uint8
  uint8_t  3 : Constant  OutDataTypeStr=uint8
  Out1 : Outport
  wires:
  Read Bit Set/1 -> Mux/1  "Addres/RW Byte euler_heading Teensy Status will be returned here"
  Inport/1 -> Read Bit Set/1
  uint8_t  3/1 -> Mux/4  "Byte 1 will be returned here"
  Mux/1 -> Out1/1
  uint8_t  2/1 -> Mux/3  "Byte 0 will be returned here"
  uint8_t  1/1 -> Mux/2  "Junk will be returned here"

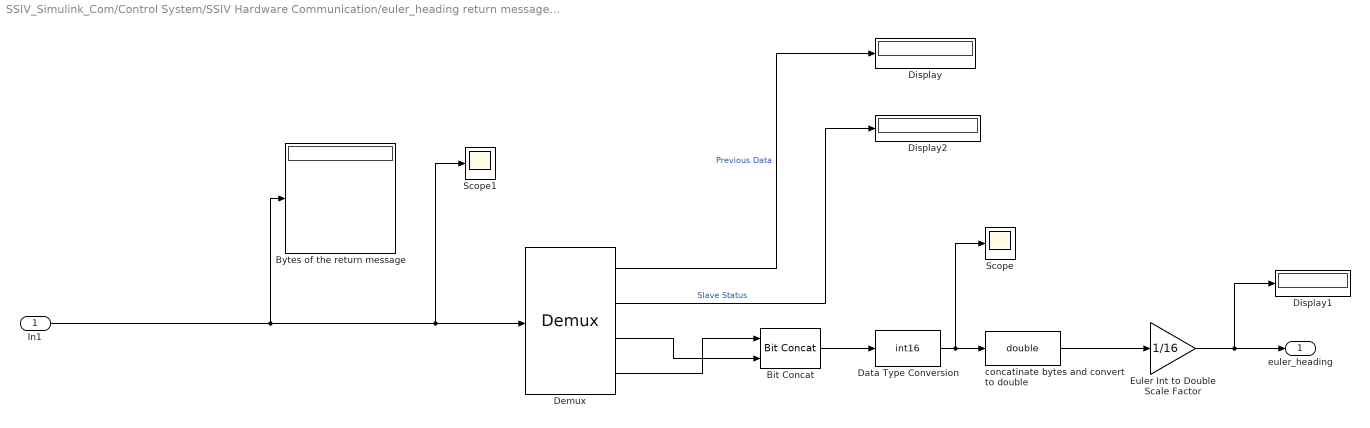
== system SSIV_Simulink_Com/Control System/SSIV Hardware Communication/euler_heading return message (Slave --> Master) ==
  In1 : Inport
  Bit Concat : hdlsllib/Logic and Bit Operations/Bit Concat  numInputs=2
      settings: SourceProductName=HDL Coder  SourceProductBaseCode=HD
  Bytes of the return message : Display
      settings: Format=decimal (Stored Integer)
  Data Type Conversion : DataTypeConversion  OutDataTypeStr=int16  RndMeth=Nearest
  Demux : Demux
  Display : Display
      settings: Format=binary (Stored Integer)
  Display1 : Display
      settings: Format=decimal (Stored Integer)
  Display2 : Display
      settings: Format=binary (Stored Integer)
  Euler Int to Double Scale Factor : Gain  Gain=1/16
  Scope : Scope
  Scope1 : Scope
  concatinate bytes and convert to double : DataTypeConversion  OutDataTypeStr=double  RndMeth=Nearest  LockScale=on
  euler_heading : Outport
  wires:
  concatinate bytes and convert to double/1 -> Euler Int to Double Scale Factor/1
  Demux/2 -> Display2/1  "Slave Status"
  Demux/1 -> Display/1  "Previous Data"
  In1/1 -> Bytes of the return message/1, Scope1/1, Demux/1
  Demux/4 -> Bit Concat/1
  Demux/3 -> Bit Concat/2
  Euler Int to Double Scale Factor/1 -> Display1/1, euler_heading/1
  Bit Concat/1 -> Data Type Conversion/1
  Data Type Conversion/1 -> Scope/1, concatinate bytes and convert to double/1

== system SSIV_Simulink_Com/Control System/SSIV Hardware Communication/euler_pitch read message (Master --> Slave) ==
  Inport : Inport
  Mux : Mux
      settings: DisplayOption=signals
  Read Bit Set : simulink/Logic and Bit Operations/Bit Set  iBit=7
      settings: SourceProductName=Simulink  SourceProductBaseCode=SL
  uint8_t 1 : Constant  OutDataTypeStr=uint8
  uint8_t 2 : Constant  OutDataTypeStr=uint8
  uint8_t 3 : Constant  OutDataTypeStr=uint8
  Out1 : Outport
  wires:
  Read Bit Set/1 -> Mux/1  "Addres/RW Byte euler_pitch Teensy Status will be returned here"
  uint8_t 1/1 -> Mux/2  "Junk will be returned here"
  Inport/1 -> Read Bit Set/1
  uint8_t 3/1 -> Mux/4  "Byte 1 will be returned here"
  Mux/1 -> Out1/1
  uint8_t 2/1 -> Mux/3  "Byte 0 will be returned here"

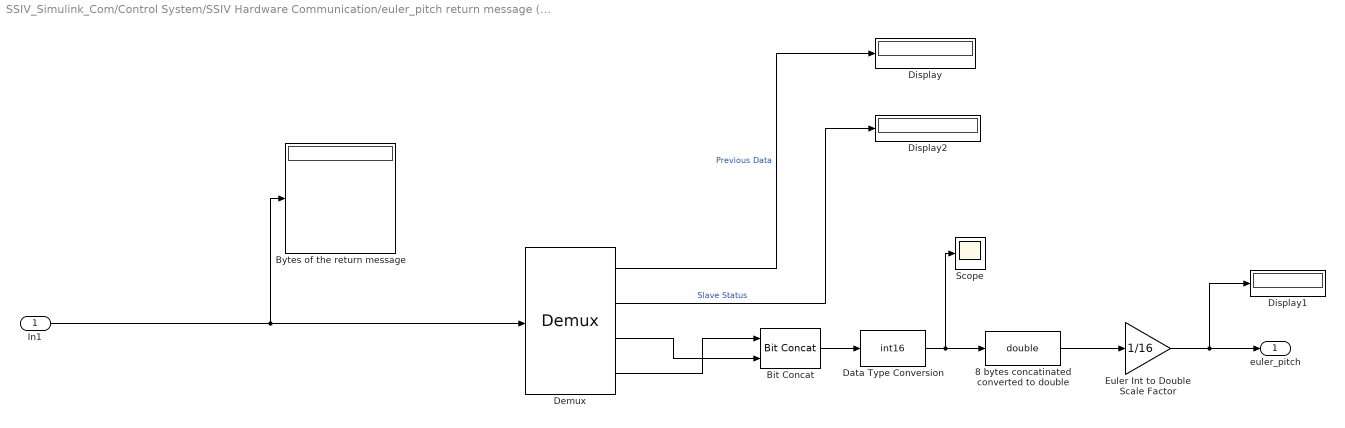
== system SSIV_Simulink_Com/Control System/SSIV Hardware Communication/euler_pitch return message (Slave --> Master) ==
  In1 : Inport
  8 bytes concatinated converted to double : DataTypeConversion  OutDataTypeStr=double  RndMeth=Nearest
  Bit Concat : hdlsllib/Logic and Bit Operations/Bit Concat  numInputs=2
      settings: SourceProductName=HDL Coder  SourceProductBaseCode=HD
  Bytes of the return message : Display
      settings: Format=decimal (Stored Integer)
  Data Type Conversion : DataTypeConversion  OutDataTypeStr=int16
  Demux : Demux
  Display : Display
      settings: Format=binary (Stored Integer)
  Display1 : Display
      settings: Format=decimal (Stored Integer)
  Display2 : Display
      settings: Format=binary (Stored Integer)
  Euler Int to Double Scale Factor : Gain  Gain=1/16  SaturateOnIntegerOverflow=on
  Scope : Scope
  euler_pitch : Outport
  wires:
  8 bytes concatinated converted to double/1 -> Euler Int to Double Scale Factor/1
  Demux/2 -> Display2/1  "Slave Status"
  Demux/1 -> Display/1  "Previous Data"
  In1/1 -> Bytes of the return message/1, Demux/1
  Bit Concat/1 -> Data Type Conversion/1
  Demux/4 -> Bit Concat/1
  Demux/3 -> Bit Concat/2
  Euler Int to Double Scale Factor/1 -> Display1/1, euler_pitch/1
  Data Type Conversion/1 -> Scope/1, 8 bytes concatinated converted to double/1

== system SSIV_Simulink_Com/Control System/SSIV Hardware Communication/euler_roll read message (Master --> Slave) ==
  Inport : Inport
  Mux : Mux
      settings: DisplayOption=signals
  Read Bit Set : simulink/Logic and Bit Operations/Bit Set  iBit=7
      settings: SourceProductName=Simulink  SourceProductBaseCode=SL
  uint8_t  1 : Constant  OutDataTypeStr=uint8
  uint8_t  2 : Constant  OutDataTypeStr=uint8
  uint8_t  3 : Constant  OutDataTypeStr=uint8
  Out1 : Outport
  wires:
  Read Bit Set/1 -> Mux/1  "Addres/RW Byte euler_roll Teensy Status will be returned here"
  Inport/1 -> Read Bit Set/1
  uint8_t  3/1 -> Mux/4  "Byte 1 will be returned here"
  Mux/1 -> Out1/1
  uint8_t  2/1 -> Mux/3  "Byte 0 will be returned here"
  uint8_t  1/1 -> Mux/2  "Junk will be returned here"

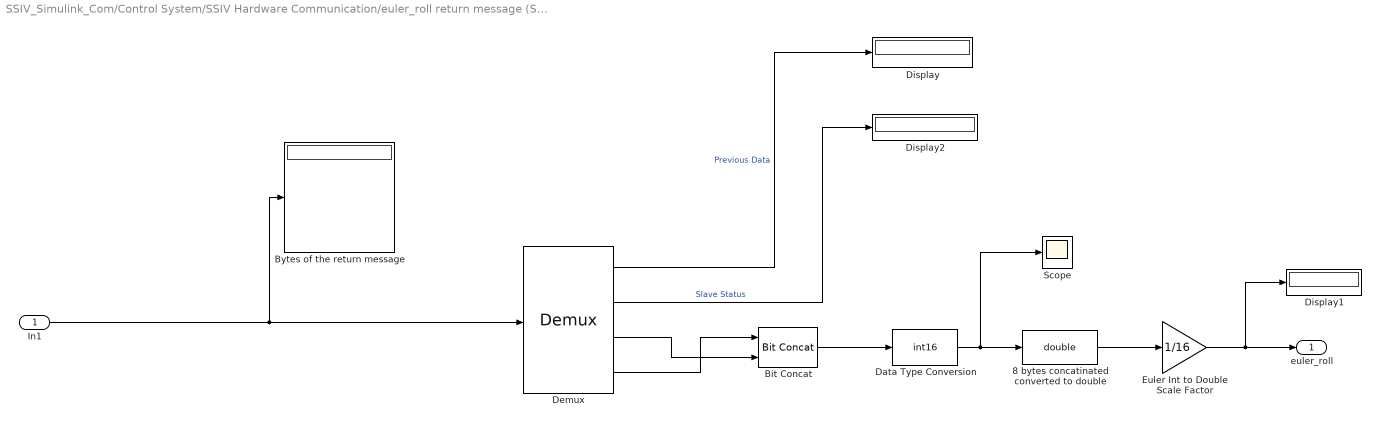
== system SSIV_Simulink_Com/Control System/SSIV Hardware Communication/euler_roll return message (Slave --> Master) ==
  In1 : Inport
  8 bytes concatinated converted to double : DataTypeConversion  OutDataTypeStr=double  RndMeth=Nearest
  Bit Concat : hdlsllib/Logic and Bit Operations/Bit Concat  numInputs=2
      settings: SourceProductName=HDL Coder  SourceProductBaseCode=HD
  Bytes of the return message : Display
      settings: Format=decimal (Stored Integer)
  Data Type Conversion : DataTypeConversion  OutDataTypeStr=int16  RndMeth=Nearest
  Demux : Demux
  Display : Display
      settings: Format=binary (Stored Integer)
  Display1 : Display
      settings: Format=decimal (Stored Integer)
  Display2 : Display
      settings: Format=binary (Stored Integer)
  Euler Int to Double Scale Factor : Gain  Gain=1/16
  Scope : Scope
  euler_roll : Outport
  wires:
  8 bytes concatinated converted to double/1 -> Euler Int to Double Scale Factor/1
  Demux/2 -> Display2/1  "Slave Status"
  Demux/1 -> Display/1  "Previous Data"
  In1/1 -> Bytes of the return message/1, Demux/1
  Bit Concat/1 -> Data Type Conversion/1
  Demux/4 -> Bit Concat/1
  Demux/3 -> Bit Concat/2
  Euler Int to Double Scale Factor/1 -> Display1/1, euler_roll/1
  Data Type Conversion/1 -> Scope/1, 8 bytes concatinated converted to double/1

== system SSIV_Simulink_Com/Control System/SSIV Hardware Communication/gyr_x read message (Master --> Slave) ==
  Inport : Inport
  Mux : Mux
      settings: DisplayOption=signals
  Read Bit Set : simulink/Logic and Bit Operations/Bit Set  iBit=7
      settings: SourceProductName=Simulink  SourceProductBaseCode=SL
  uint8_t 1 : Constant  OutDataTypeStr=uint8
  uint8_t 2 : Constant  OutDataTypeStr=uint8
  uint8_t 3 : Constant  OutDataTypeStr=uint8
  Out1 : Outport
  wires:
  uint8_t 2/1 -> Mux/3  "Byte 0 will be returned here"
  Mux/1 -> Out1/1
  uint8_t 3/1 -> Mux/4  "Byte 1 will be returned here"
  Inport/1 -> Read Bit Set/1
  uint8_t 1/1 -> Mux/2  "Junk will be returned here"
  Read Bit Set/1 -> Mux/1  "Addres/RW Byte gyr_x Teensy Status will be returned here"

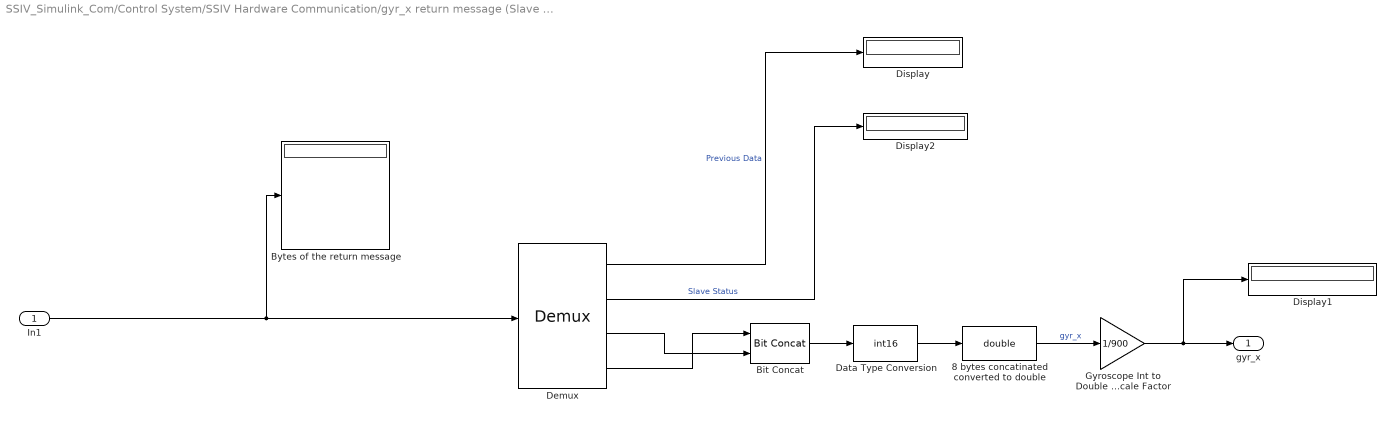
== system SSIV_Simulink_Com/Control System/SSIV Hardware Communication/gyr_x return message (Slave --> Master) ==
  In1 : Inport
  8 bytes concatinated converted to double : DataTypeConversion  OutDataTypeStr=double  RndMeth=Nearest
  Bit Concat : hdlsllib/Logic and Bit Operations/Bit Concat  numInputs=2
      settings: SourceProductName=HDL Coder  SourceProductBaseCode=HD
  Bytes of the return message : Display
      settings: Format=decimal (Stored Integer)
  Data Type Conversion : DataTypeConversion  OutDataTypeStr=int16  RndMeth=Nearest
  Demux : Demux
  Display : Display
      settings: Format=binary (Stored Integer)
  Display1 : Display
      settings: Format=decimal (Stored Integer)
  Display2 : Display
      settings: Format=binary (Stored Integer)
  Gyroscope Int to Double Scale Factor : Gain  Gain=1/900
  gyr_x : Outport
  wires:
  Gyroscope Int to Double Scale Factor/1 -> gyr_x/1, Display1/1
  Demux/3 -> Bit Concat/2
  Demux/4 -> Bit Concat/1
  Bit Concat/1 -> Data Type Conversion/1
  In1/1 -> Demux/1, Bytes of the return message/1
  Demux/1 -> Display/1  "Previous Data"
  Demux/2 -> Display2/1  "Slave Status"
  8 bytes concatinated converted to double/1 -> Gyroscope Int to Double Scale Factor/1  "gyr_x"
  Data Type Conversion/1 -> 8 bytes concatinated converted to double/1

== system SSIV_Simulink_Com/Control System/SSIV Hardware Communication/gyr_y read message (Master --> Slave) ==
  Inport : Inport
  Mux : Mux
      settings: DisplayOption=signals
  Read Bit Set : simulink/Logic and Bit Operations/Bit Set  iBit=7
      settings: SourceProductName=Simulink  SourceProductBaseCode=SL
  uint8_t 1 : Constant  OutDataTypeStr=uint8
  uint8_t 2 : Constant  OutDataTypeStr=uint8
  uint8_t 3 : Constant  OutDataTypeStr=uint8
  Out1 : Outport
  wires:
  Read Bit Set/1 -> Mux/1  "Addres/RW Byte gyr_y Teensy Status will be returned here"
  uint8_t 1/1 -> Mux/2  "Junk will be returned here"
  Inport/1 -> Read Bit Set/1
  uint8_t 3/1 -> Mux/4  "Byte 1 will be returned here"
  Mux/1 -> Out1/1
  uint8_t 2/1 -> Mux/3  "Byte 0 will be returned here"

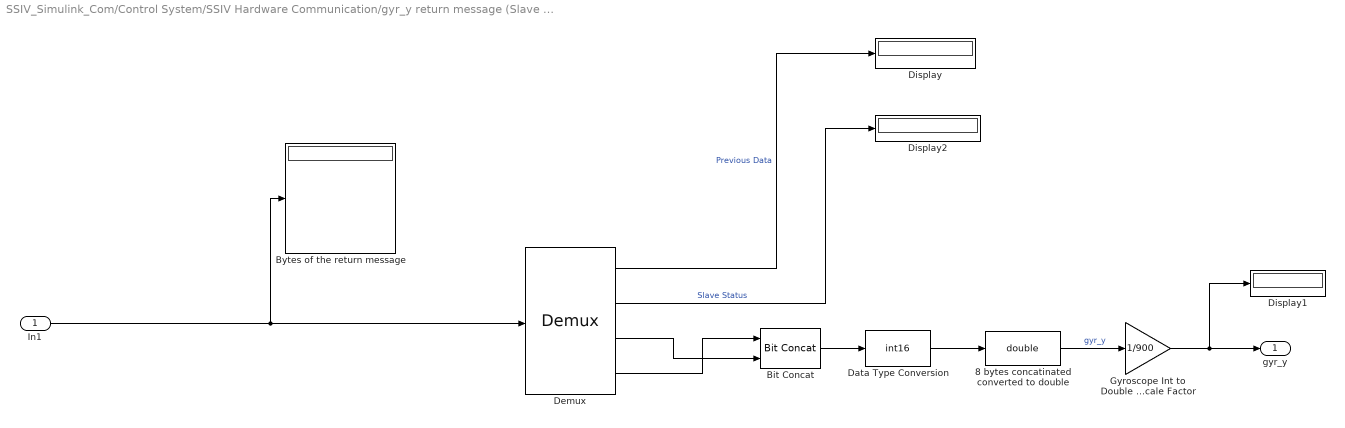
== system SSIV_Simulink_Com/Control System/SSIV Hardware Communication/gyr_y return message (Slave --> Master) ==
  In1 : Inport
  8 bytes concatinated converted to double : DataTypeConversion  OutDataTypeStr=double  RndMeth=Nearest
  Bit Concat : hdlsllib/Logic and Bit Operations/Bit Concat  numInputs=2
      settings: SourceProductName=HDL Coder  SourceProductBaseCode=HD
  Bytes of the return message : Display
      settings: Format=decimal (Stored Integer)
  Data Type Conversion : DataTypeConversion  OutDataTypeStr=int16  RndMeth=Nearest
  Demux : Demux
  Display : Display
      settings: Format=binary (Stored Integer)
  Display1 : Display
      settings: Format=decimal (Stored Integer)
  Display2 : Display
      settings: Format=binary (Stored Integer)
  Gyroscope Int to Double Scale Factor : Gain  Gain=1/900
  gyr_y : Outport
  wires:
  8 bytes concatinated converted to double/1 -> Gyroscope Int to Double Scale Factor/1  "gyr_y"
  Demux/2 -> Display2/1  "Slave Status"
  Demux/1 -> Display/1  "Previous Data"
  In1/1 -> Bytes of the return message/1, Demux/1
  Bit Concat/1 -> Data Type Conversion/1
  Demux/4 -> Bit Concat/1
  Demux/3 -> Bit Concat/2
  Gyroscope Int to Double Scale Factor/1 -> Display1/1, gyr_y/1
  Data Type Conversion/1 -> 8 bytes concatinated converted to double/1

== system SSIV_Simulink_Com/Control System/SSIV Hardware Communication/gyr_z read message (Master --> Slave) ==
  Inport : Inport
  Mux : Mux
      settings: DisplayOption=signals
  Read Bit Set : simulink/Logic and Bit Operations/Bit Set  iBit=7
      settings: SourceProductName=Simulink  SourceProductBaseCode=SL
  uint8_t 1 : Constant  OutDataTypeStr=uint8
  uint8_t 2 : Constant  OutDataTypeStr=uint8
  uint8_t 3 : Constant  OutDataTypeStr=uint8
  Out1 : Outport
  wires:
  uint8_t 2/1 -> Mux/3  "Byte 0 will be returned here"
  Mux/1 -> Out1/1
  uint8_t 3/1 -> Mux/4  "Byte 1 will be returned here"
  Inport/1 -> Read Bit Set/1
  uint8_t 1/1 -> Mux/2  "Junk will be returned here"
  Read Bit Set/1 -> Mux/1  "Addres/RW Byte gyr_z Teensy Status will be returned here"

== system SSIV_Simulink_Com/Control System/SSIV Hardware Communication/gyr_z return message (Slave --> Master) ==
  In1 : Inport
  8 bytes concatinated converted to double : DataTypeConversion  OutDataTypeStr=double
  Bit Concat : hdlsllib/Logic and Bit Operations/Bit Concat  numInputs=2
      settings: SourceProductName=HDL Coder  SourceProductBaseCode=HD
  Bytes of the return message : Display
      settings: Format=decimal (Stored Integer)
  Data Type Conversion : DataTypeConversion  OutDataTypeStr=int16  RndMeth=Nearest
  Demux : Demux
  Display : Display
      settings: Format=binary (Stored Integer)
  Display1 : Display
      settings: Format=decimal (Stored Integer)
  Display2 : Display
      settings: Format=binary (Stored Integer)
  Gyroscope Int to Double Scale Factor : Gain  Gain=1/900
  gyr_z : Outport
  wires:
  Gyroscope Int to Double Scale Factor/1 -> gyr_z/1, Display1/1
  Demux/3 -> Bit Concat/2
  Demux/4 -> Bit Concat/1
  Bit Concat/1 -> Data Type Conversion/1
  In1/1 -> Demux/1, Bytes of the return message/1
  Demux/1 -> Display/1  "Previous Data"
  Demux/2 -> Display2/1  "Slave Status"
  8 bytes concatinated converted to double/1 -> Gyroscope Int to Double Scale Factor/1  "gyr_z"
  Data Type Conversion/1 -> 8 bytes concatinated converted to double/1

== system SSIV_Simulink_Com/Control System/SSIV Hardware Communication/radio_steering read message (Master --> Slave) ==
  Inport : Inport
  Mux : Mux
      settings: DisplayOption=signals
  Read Bit Set : simulink/Logic and Bit Operations/Bit Set  iBit=7
      settings: SourceProductName=Simulink  SourceProductBaseCode=SL
  uint8_t 1 : Constant  OutDataTypeStr=uint8
  uint8_t 2 : Constant  OutDataTypeStr=uint8
  uint8_t 3 : Constant  OutDataTypeStr=uint8
  Out1 : Outport
  wires:
  Read Bit Set/1 -> Mux/1  "Addres/RW Byte radio_steering Teensy Status will be returned here"
  uint8_t 1/1 -> Mux/2  "Junk will be returned here"
  Inport/1 -> Read Bit Set/1
  uint8_t 3/1 -> Mux/4  "Byte 1 will be returned here"
  Mux/1 -> Out1/1
  uint8_t 2/1 -> Mux/3  "Byte 0 will be returned here"

== system SSIV_Simulink_Com/Control System/SSIV Hardware Communication/radio_steering return message (Slave --> Master) ==
  In1 : Inport
  8 bytes concatinated converted to double : DataTypeConversion  OutDataTypeStr=double  RndMeth=Nearest
  Bit Concat : hdlsllib/Logic and Bit Operations/Bit Concat  numInputs=2
      settings: SourceProductName=HDL Coder  SourceProductBaseCode=HD
  Bytes of the return message : Display
      settings: Format=decimal (Stored Integer)
  Data Type Conversion : DataTypeConversion  OutDataTypeStr=int16  RndMeth=Nearest
  Demux : Demux
  Display : Display
      settings: Format=binary (Stored Integer)
  Display1 : Display
      settings: Format=decimal (Stored Integer)
  Display2 : Display
      settings: Format=binary (Stored Integer)
  radio_steering : Outport
  wires:
  8 bytes concatinated converted to double/1 -> Display1/1, radio_steering/1  "radio_steering"
  Demux/2 -> Display2/1  "Slave Status"
  Demux/1 -> Display/1  "Previous Data"
  In1/1 -> Bytes of the return message/1, Demux/1
  Bit Concat/1 -> Data Type Conversion/1
  Demux/4 -> Bit Concat/1
  Demux/3 -> Bit Concat/2
  Data Type Conversion/1 -> 8 bytes concatinated converted to double/1

== system SSIV_Simulink_Com/Control System/SSIV Hardware Communication/radio_throttle read message (Master --> Slave) ==
  Inport : Inport
  Mux : Mux
      settings: DisplayOption=signals
  Read Bit Set : simulink/Logic and Bit Operations/Bit Set  iBit=7
      settings: SourceProductName=Simulink  SourceProductBaseCode=SL
  uint8_t 1 : Constant  OutDataTypeStr=uint8
  uint8_t 2 : Constant  OutDataTypeStr=uint8
  uint8_t 3 : Constant  OutDataTypeStr=uint8
  Out1 : Outport
  wires:
  Read Bit Set/1 -> Mux/1  "Addres/RW Byte radio_throttle Teensy Status will be returned here"
  uint8_t 1/1 -> Mux/2  "Junk will be returned here"
  Inport/1 -> Read Bit Set/1
  uint8_t 3/1 -> Mux/4  "Byte 1 will be returned here"
  Mux/1 -> Out1/1
  uint8_t 2/1 -> Mux/3  "Byte 0 will be returned here"

== system SSIV_Simulink_Com/Control System/SSIV Hardware Communication/radio_throttle return message (Slave --> Master) ==
  In1 : Inport
  8 bytes concatinated converted to double : DataTypeConversion  OutDataTypeStr=double  RndMeth=Nearest
  Bit Concat : hdlsllib/Logic and Bit Operations/Bit Concat  numInputs=2
      settings: SourceProductName=HDL Coder  SourceProductBaseCode=HD
  Bytes of the return message : Display
      settings: Format=decimal (Stored Integer)
  Data Type Conversion : DataTypeConversion  OutDataTypeStr=int16  RndMeth=Nearest
  Demux : Demux
  Display : Display
      settings: Format=binary (Stored Integer)
  Display1 : Display
      settings: Format=decimal (Stored Integer)
  Display2 : Display
      settings: Format=binary (Stored Integer)
  radio_throttle : Outport
  wires:
  8 bytes concatinated converted to double/1 -> Display1/1, radio_throttle/1  "radio_throttle"
  Demux/2 -> Display2/1  "Slave Status"
  Demux/1 -> Display/1  "Previous Data"
  In1/1 -> Bytes of the return message/1, Demux/1
  Bit Concat/1 -> Data Type Conversion/1
  Demux/4 -> Bit Concat/1
  Demux/3 -> Bit Concat/2
  Data Type Conversion/1 -> 8 bytes concatinated converted to double/1

== system SSIV_Simulink_Com/Control System/SSIV Hardware Communication/servo_out Write Message (Master --> Slave) ==
  In1 : Inport
  Bit Slice2 : hdlsllib/Logic and Bit Operations/Bit Slice  lidx=15  ridx=8
  Bit Slice3 : hdlsllib/Logic and Bit Operations/Bit Slice  lidx=7  ridx=0
  Display5 : Display
      settings: Format=decimal (Stored Integer)
  Mux : Mux  Inputs=2
      settings: DisplayOption=signals
  Out1 : Outport
  wires:
  In1/1 -> Display5/1, Bit Slice3/1, Bit Slice2/1  "Servo"
  Mux/1 -> Out1/1
  Bit Slice3/1 -> Mux/1
  Bit Slice2/1 -> Mux/2
